simulink model "HW6_Inv_sim_2_wFriction"  (R2015b)
settings: Solver=ode3  StartTime=0.0  StopTime=5  FixedStep=0.001  RelTol=1e-3
values from neighbouring files (symbols this model uses):
  F = [120  22 20 28]    [HW6_InvP_cntrl_1_wFriction.m]
  u_sat = 80    [HW6_InvP_cntrl_1_wFriction.m]
  x1_0 = x1_0_deg*3.1416/180    (= 0.2618)    [HW6_InvP_cntrl_1_wFriction.m]
  x3_0 = 0.2    [HW6_InvP_cntrl_1_wFriction.m]
settings Model: ExtModeTrigMode=oneshot  ExtModeArmWhenConnect=off  Creator=BC  LastModifiedBy=bcc88
settings DataIOCC: LimitDataPoints=off  SaveFormat=Array  SignalLoggingSaveFormat=ModelDataLogs
settings OptimizationCC: BlockReduction=off  BooleanDataType=off  ExpressionDepthLimit=2147483647  InitFltsAndDblsToZero=on
settings DebuggingCC: SaveWithParameterizedLinksMsg=none  UnderspecifiedInitializationDetection=Classic  MergeDetectMultiDrivingBlocksExec=none  SignalResolutionControl=TryResolveAllWithWarning  MultiTaskDSMMsg=warning  MultiTaskCondExecSysMsg=none  FcnCallInpInsideContextMsg=UseLocalSettings  StateNameClashWarn=warning
settings HardwareCC: ProdBitPerPointer=32  ProdLargestAtomicFloat=None  ProdIntDivRoundTo=Undefined  ProdEndianess=Unspecified  ProdWordSize=32  ProdHWDeviceType=32-bit Generic  TargetUnknown=on
settings GRTTargetCC: TargetFcnLib=ansi_tfl_tmw.mat  CombineOutputUpdateFcns=off  GRTInterface=on
settings ConfigComp: CovModelRefEnable=Off

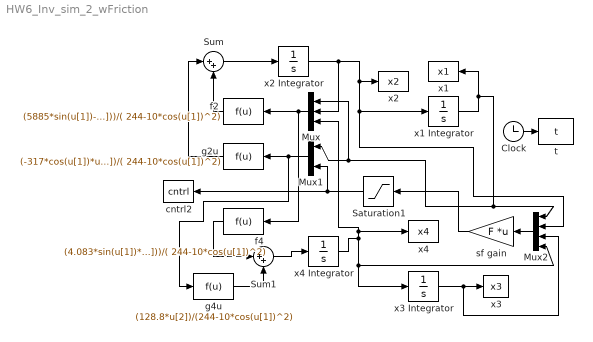
== system HW6_Inv_sim_2_wFriction ==
  Clock : Clock
  Mux : Mux  Inputs=3
  Mux1 : Mux  Inputs=2
  Mux2 : Mux
  Saturation1 : Saturate  UpperLimit=u_sat  LowerLimit=-u_sat
  Sum : Sum  Inputs=|++
  Sum1 : Sum  Inputs=|++
  cntrl2 : ToWorkspace  VariableName=cntrl  SampleTime=-1
  f2 : Fcn  Expr=(5885*sin(u[1])-10*sin(u[1])*cos(u[1])*u[2]^2-378.8*u[2] +79.25*u[3]*cos(u[1]))/( 244-10*cos(u[1])^2)
  f4 : Fcn  Expr=(4.083*sin(u[1])*u[2]^2-32.2*u[3]- 98.5*sin(u[1])*cos(u[1])+6.34*u[2]*cos(u[1]))/( 244-10*cos(u[1])^2)
  g2u : Fcn  Expr=(-317*cos(u[1])*u[2])/( 244-10*cos(u[1])^2)
  g4u : Fcn  Expr=(128.8*u[2])/(244-10*cos(u[1])^2)
  sf gain : Gain  Gain=F  Multiplication=Matrix(K*u)
  t : ToWorkspace  VariableName=t  SampleTime=-1
  x1 : ToWorkspace  VariableName=x1  SampleTime=-1
  x1 Integrator : Integrator  InitialCondition=x1_0
  x2 : ToWorkspace  VariableName=x2  SampleTime=-1
  x2 Integrator : Integrator
  x3 : ToWorkspace  VariableName=x3  SampleTime=-1
  x3 Integrator : Integrator  InitialCondition=x3_0
  x4 : ToWorkspace  VariableName=x4  SampleTime=-1
  x4 Integrator : Integrator
  wires:
  x2 Integrator/1 -> x1 Integrator/1, Mux2/2, x2/1, Mux/2
  Clock/1 -> t/1
  Mux/1 -> f2/1, f4/1
  f2/1 -> Sum/2
  Sum/1 -> x2 Integrator/1
  g2u/1 -> Sum/1
  Mux1/1 -> g2u/1, g4u/1
  Mux2/1 -> sf gain/1
  x3 Integrator/1 -> Mux2/3, x3/1
  Sum1/1 -> x4 Integrator/1
  f4/1 -> Sum1/1
  x4 Integrator/1 -> x4/1, Mux/3, x3 Integrator/1, Mux2/4
  g4u/1 -> Sum1/2
  sf gain/1 -> Saturation1/1
  x1 Integrator/1 -> x1/1, Mux/1, Mux1/1, Mux2/1
  Saturation1/1 -> cntrl2/1, Mux1/2
